simulink model "TASK1_regulation"  (R2024b)
settings: Solver=FixedStepAuto  StartTime=0.0  StopTime=inf  RelTol=1e-3
values from neighbouring files (symbols this model uses):
  D = diag([0.001, 0.001, 0.001, 0.0175/6, 0.0175/6, 0.0175/6*T_s, 0.0175/6*T_s].^2)    [TASK1_init_regulation.m]    (also in init_regulation.m)
  d = d_nominal    (= 0.165)    [TASK1_init_regulation.m]    (also in init_regulation.m)
  d_actual = d_nominal    (= 0.165)    [TASK1_init_regulation.m]    (also in init_regulation.m)
  omega_M = 10    [TASK1_init_regulation.m]    (also in init_regulation.m)
  P_INIT_EKF = diag([0.101, 0.101, 0.101, 0.0175/6, 0.0175/6, 0.0175/6*T_s, 0.0175/6*T_s].^2)    [TASK1_init_regulation.m]    (also in init_regulation.m = diag([0.001, 0.001, 0.001, 0.0175/6, 0.0175/6, 0.0175/6*T_s,)
  p_loss = 0    [TASK1_init_regulation.m]    (also in init_regulation.m)
  q_d = [x(2);y(2);0]    [TASK1_init_regulation.m]    (also in init_regulation.m = [2;2;0])
  Q_INIT = [x(1)+0.5;y(8)-0.5;-pi/2]    [TASK1_init_regulation.m]    (also in init_regulation.m = [0;0;0])
  r = r_nominal    (= 0.03)    [TASK1_init_regulation.m]    (also in init_regulation.m)
  R_2 = diag([ENCODER_QUANTIZATION/6,ENCODER_QUANTIZATION/6].^2)    [TASK1_init_regulation.m]    (also in init_regulation.m)
  R_3 = diag(([0.001, ENCODER_QUANTIZATION/6,ENCODER_QUANTIZATION/6]).^2)    [TASK1_init_regulation.m]    (also in init_regulation.m)
  R_4 = diag(([0.001, 0.001, ENCODER_QUANTIZATION/6,ENCODER_QUANTIZATION/6]).^2)    [TASK1_init_regulation.m]    (also in init_regulation.m)
  R_5 = diag(([0.001, 0.001, 0.001, ENCODER_QUANTIZATION/6,ENCODER_QUANTIZATION/6]).^2)    [TASK1_init_regulation.m]    (also in init_regulation.m)
  r_actual = r_nominal    (= 0.03)    [TASK1_init_regulation.m]    (also in init_regulation.m)
  T_s = 0.04    [TASK1_init_regulation.m]    (also in init_regulation.m)
  Z_INIT_EKF = [Q_INIT; 0; 0; 0; 0]    [TASK1_init_regulation.m]    (also in init_regulation.m)
undefined symbols (not defined in the file or in its folder): X, Y
libraries: robotlib x6, sharedtransform x1, dspsigops x1
settings Model: SimulationMode=external  Creator=riccardo01  LastModifiedBy=defendenri
settings DataIOCC: SaveFormat=Array  ReturnWorkspaceOutputs=off
settings OptimizationCC: DefaultParameterBehavior=Inlined  EnhancedBackFolding=on  PassReuseOutputArgsAs=Individual arguments  ZeroExternalMemoryAtStartup=off  ZeroInternalMemoryAtStartup=off  MaxStackSize=64  OptimizeBlockOrder=speed  DifferentSizesBufferReuse=on  OptimizationCustomize=off  EfficientTunableParamExpr=on
settings DebuggingCC: AlgebraicLoopMsg=none  ParameterTunabilityLossMsg=error
settings HardwareCC: ProdBitPerPointer=32  ProdBitPerSizeT=32  ProdBitPerPtrDiffT=32  ProdLargestAtomicFloat=None  ProdIntDivRoundTo=Undefined  ProdEndianess=Unspecified  ProdWordSize=32  ProdHWDeviceType=Generic->Unspecified (assume 32-bit Generic)
settings SFSimCC: MATLABDynamicMemAlloc=off
settings RTWCC: Description=Embedded Coder  SystemTargetFile=ert.tlc  HardwareBoard=Robot Operating System (ROS)  TLCOptions="-aInlineSetEventsForThisBaseRateFcn=TLC_FALSE -aSuppressMultiTaskScheduler=TLC_FALSE  -aRateBasedStepFcn=0"  TemplateMakefile=ert_default_tmf  Toolchain=Catkin  TargetLang=C++
settings CodeAppCC: ForceParamTrailComments=on  IgnoreCustomStorageClasses=off  OperatorAnnotations=on  SimulinkDataObjDesc=on  SFDataObjDesc=on  InsertBlockDesc=on

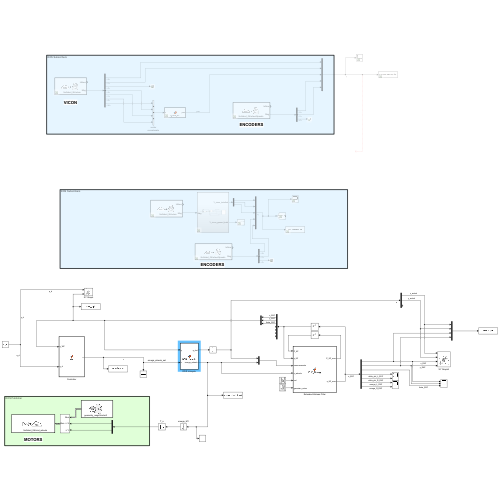
[thumbnail: Simulink's stored preview of the top-level diagram]
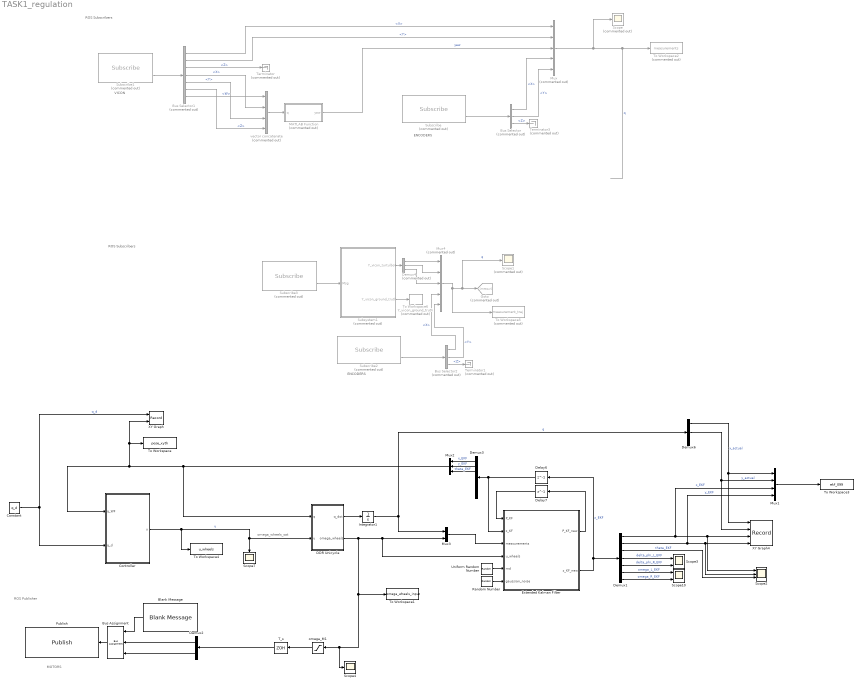
== system TASK1_regulation ==
  note: MOTORS
  note: ROS Publisher
  note: ENCODERS
  note: VICON
  note: ROS Subscribers
  note: omega_wheels_sat
  note: ENCODERS
  note: ROS Subscribers
  Blank Message : robotlib/Blank Message  messageClass=Message  entityType=geometry_msgs/Vector3  messageType=geometry_msgs/Vector3  SampleTime=T_s  legacyBusStruct=off
      settings: LibrarySourceBlock=roslib/ROS/Blank Message
  Bus Assignment : BusAssignment  AssignedSignals=X,Y
  Bus Selector : BusSelector  Commented=on  OutputSignals=X,Y,Z
  Bus Selector1 : BusSelector  Commented=on  OutputSignals=Pose.Pose.Position.X,Pose.Pose.Position.Y,Pose.Pose.Position.Z,Pose.Pose.Orientation.X,Pose.Pose.Orientation.Y,Pose.Pose.Orientation.Z,Pose.Pose.Orientation.W
  Bus Selector2 : BusSelector  Commented=on  OutputSignals=X,Y,Z
  Constant : Constant  Value=q_d
  Controller : MATLAB Function  TreatAsAtomicUnit=on
  DDR Unicycle : MATLAB Function  TreatAsAtomicUnit=on
  Delay6 : Delay  DelayLength=1  InitialCondition=Z_INIT_EKF  SampleTime=T_s
  Delay7 : Delay  DelayLength=1  InitialCondition=P_INIT_EKF  SampleTime=T_s
  Demux1 : Demux  Outputs=7
  Demux2 : Demux  Outputs=2
  Demux3 : Demux  Outputs=7
  Demux4 : Demux  Commented=on  Outputs=3
  Demux6 : Demux  Outputs=3
  Extended Kalman Filter : MATLAB Function  TreatAsAtomicUnit=on
  Goto : Goto  Commented=on  GotoTag=measur
  Integrator1 : Integrator  InitialCondition=Q_INIT
  MATLAB Function : MATLAB Function  Commented=on  TreatAsAtomicUnit=on
  Mux : Mux  Commented=on  Inputs=5
  Mux1 : Mux
  Mux2 : Mux  Inputs=3
  Mux3 : Mux  Inputs=2
  Mux4 : Mux  Commented=on  Inputs=5
  Publish : robotlib/Publish  topicSource=Specify your own  topic=/turtlebot_06/cmd_wheels  messageType=geometry_msgs/Vector3  legacyBusStruct=off  messageQueueLength=1
      settings: LibrarySourceBlock=roslib/ROS/Publish
  Random Number : RandomNumber  Variance=0.01  SampleTime=T_s
  Scope : Scope  Commented=on
  Scope1 : Scope  Commented=on
  Scope10 : Scope  NumInputPorts=2
  Scope2 : Scope  NumInputPorts=3
  Scope3 : Scope  NumInputPorts=2
  Scope4 : Scope
  Scope7 : Scope
  Subscribe : robotlib/Subscribe  Commented=on  topicSource=Specify your own  topic=/turtlebot_06/wheelSpeeds  messageType=geometry_msgs/Vector3  SampleTime=T_s  legacyBusStruct=off  messageQueueLength=1
      settings: LibrarySourceBlock=roslib/ROS/Subscribe
  Subscribe1 : robotlib/Subscribe  Commented=on  topicSource=Specify your own  topic=/turtlebot_06/odom  messageType=nav_msgs/Odometry  SampleTime=T_s  legacyBusStruct=off  messageQueueLength=1
      settings: LibrarySourceBlock=roslib/ROS/Subscribe
  Subscribe2 : robotlib/Subscribe  Commented=on  topicSource=Specify your own  topic=/turtlebot_06/wheelSpeeds  messageType=geometry_msgs/Vector3  SampleTime=T_s  legacyBusStruct=off  messageQueueLength=1
      settings: LibrarySourceBlock=roslib/ROS/Subscribe
  Subscribe3 : robotlib/Subscribe  Commented=on  topicSource=Specify your own  topic=/turtlebot_06/odom  messageType=nav_msgs/Odometry  SampleTime=T_s  legacyBusStruct=off  messageQueueLength=1
      settings: LibrarySourceBlock=roslib/ROS/Subscribe
  Subsystem1 : Subsystem  Commented=on
  T_s : ZeroOrderHold  SampleTime=T_s
  Terminator : Terminator  Commented=on
  Terminator1 : Terminator  Commented=on
  Terminator3 : Terminator  Commented=on
  To Workspace : ToWorkspace  VariableName=pose_xyth  SampleTime=-1
  To Workspace1 : ToWorkspace  VariableName=omega_wheels_input  SampleTime=-1
  To Workspace2 : ToWorkspace  Commented=on  VariableName=measurements  SampleTime=-1
  To Workspace3 : ToWorkspace  VariableName=ekf_099  SaveFormat=Structure With Time  SampleTime=-1
  To Workspace4 : ToWorkspace  VariableName=u_wheels  SampleTime=T_s
  To Workspace5 : ToWorkspace  Commented=on  VariableName=measurement_traj  SaveFormat=Timeseries  SampleTime=-1
  To Workspace6 : ToWorkspace  Commented=on  VariableName=Y_vicon_ground_truth  SaveFormat=Timeseries  SampleTime=T_s
  Uniform Random Number : UniformRandomNumber  Minimum=0  SampleTime=T_s
  XY Graph : Record  FileSettingsInternal="{\"entries\":[{\"content\":{\"excelSettings\":{\"content\":{},\"type\":\"Streamout.ExcelSettings\"}},\"type\":\"Streamout.FileSettingStorage\",\"uuid\":\"\"}],\"packageUris\":[\"http:\\/\\/schema.mathworks.com\\/mf0\\/streamout_blocks\\/R2020a\"],\"version\":\"1.0\"}"  Layout=[1 2]  SignalsInternal="{\"entries\":[{\"content\":{\"signals\":[{\"content\":{\"blockPath\":[],\"dimensions\":[3],\"domain\":\"\",\"hasChildren\":true,\"lineColor\":\"#7e2f8e\",\"lineWidth\":2,\"port\":2,\"sid\":[\"\"],\"signalID\":1,\"signalName\":\"Mux2\"},\"type\":\"RecordBlkView.Signal\",\"uuid\":\"\"},{\"content\":{\"blockPath\":[],\"channel\":[1],\"dimensions\":[3],\"domain\":\"\",\"lineColor\":\"#ff6929\",\"lineWidth\":2,\"parentID\":1,\"port\":2,\"sid\":[\"\"],\"signalID\":2,\"signalName\":\"Mux2\"},\"type\":\"RecordBlkView.Signal\",\"uuid\":\"\"},{\"content\":{\"blockPath\":[],\"dimensions\":[3],\"domain\":\"\",\"hasChildren\":true,\"lineColor\":\"#d95319\",\"lineWidth\":2,\"port\":1,\"sid\":[\"\"],\"signalID\":3,\"signalName\":\"q_d\"},\"type\":\"RecordBlkView.Signal\",\"uuid\":\"\"},{\"content\":{\"blockPath\":[],\"channel\":[1],\"dimensions\":[3],\"domain\":\"\",\"lineColor\":\"#a2142f\",\"lineWidth\":2,\"parentID\":3,\"port\":1,\"sid\":[\"\"],\"signalID\":4,\"signalName\":\"q_d\"},\"type\":\"RecordBlkView.Signal\",\"uuid\":\"\"},{\"content\":{\"blockPath\":[],\"channel\":[2],\"dimensions\":[3],\"domain\":\"\",\"lineColor\":\"#139fff\",\"lineWidth\":2,\"parentID\":1,\"port\":2,\"sid\":[\"\"],\"signalID\":5,\"signalName\":\"Mux2\"},\"type\":\"RecordBlkView.Signal\",\"uuid\":\"\"},{\"content\":{\"blockPath\":[],\"channel\":[3],\"dimensions\":[3],\"domain\":\"\",\"lineColor\":\"#ff6929\",\"lineWidth\":2,\"parentID\":1,\"port\":2,\"sid\":[\"\"],\"signalID\":6,\"signalName\":\"Mux2\"},\"type\":\"RecordBlkView.Signal\",\"uuid\":\"\"},{\"content\":{\"blockPath\":[],\"channel\":[2],\"dimensions\":[3],\"domain\":\"\",\"lineColor\":\"#d95319\",\"lineWidth\":2,\"parentID\":3,\"port\":1,\"sid\":[\"\"],\"signalID\":7,\"signalName\":\"q_d\"},\"type\":\"RecordBlkView.Signal\",\"uuid\":\"\"},{\"content\":{\"blockPath\":[],\"channel\":[3],\"dimensions\":[3],\"domain\":\"\",\"lineColor\":\"#edb120\",\"lineWidth\":2,\"parentID\":3,\"port\":1,\"sid\":[\"\"],\"signalID\":8,\"signalName\":\"q_d\"},\"type\":\"RecordBlkView.Signal\",\"uuid\":\"\"}]},\"type\":\"RecordBlkView.InputSignals\",\"uuid\":\"\"}],\"packageUris\":[\"http:\\/\\/schema.mathworks.com\\/mf0\\/streamout_blocks\\/R2020a\"],\"version\":\"1.0\"}"  VisualizationBindings="{\"xyplotplugin\":{\"info\":[{\"series\":[],\"subplotID\":1}]}}"  CompatibilityTag=XY
  XY Graph4 : Record  FileSettingsInternal="{\"entries\":[{\"content\":{\"excelSettings\":{\"content\":{},\"type\":\"Streamout.ExcelSettings\"}},\"type\":\"Streamout.FileSettingStorage\",\"uuid\":\"\"}],\"packageUris\":[\"http:\\/\\/schema.mathworks.com\\/mf0\\/streamout_blocks\\/R2020a\"],\"version\":\"1.0\"}"  Layout=[1 1]  SignalsInternal="{\"entries\":[{\"content\":{\"signals\":[{\"content\":{\"blockPath\":[],\"dimensions\":[1,1],\"domain\":\"\",\"lineColor\":\"#77ac30\",\"lineWidth\":2,\"plots\":[ 1 ],\"port\":1,\"sid\":[\"\"],\"signalID\":1,\"signalName\":\"x_actual\"},\"type\":\"RecordBlkView.Signal\",\"uuid\":\"\"},{\"content\":{\"blockPath\":[],\"dimensions\":[1,1],\"domain\":\"\",\"lineColor\":\"#4dbeee\",\"lineWidth\":2,\"plots\":[ 1 ],\"port\":2,\"sid\":[\"\"],\"signalID\":2,\"signalName\":\"y_actual\"},\"type\":\"RecordBlkView.Signal\",\"uuid\":\"\"},{\"content\":{\"blockPath\":[],\"dimensions\":[1],\"domain\":\"\",\"lineColor\":\"#a2142f\",\"lineWidth\":2,\"plots\":[ 1 ],\"port\":3,\"sid\":[\"\"],\"signalID\":3,\"signalName\":\"x_EKF\"},\"type\":\"RecordBlkView.Signal\",\"uuid\":\"\"},{\"content\":{\"blockPath\":[],\"dimensions\":[1],\"domain\":\"\",\"lineColor\":\"#139fff\",\"lineWidth\":2,\"plots\":[ 1 ],\"port\":4,\"sid\":[\"\"],\"signalID\":4,\"signalName\":\"y_EKF\"},\"type\":\"RecordBlkView.Signal\",\"uuid\":\"\"}]},\"type\":\"RecordBlkView.InputSignals\",\"uuid\":\"\"}],\"packageUris\":[\"http:\\/\\/schema.mathworks.com\\/mf0\\/streamout_blocks\\/R2020a\"],\"version\":\"1.0\"}"  VisualizationBindings="{\"xyplotplugin\":{\"info\":[{\"series\":[{\"bindingParametersList\":[{\"parameter\":\"X-Axis\",\"signalID\":3,\"signalName\":\"x_EKF\"},{\"parameter\":\"Y-Axis\",\"signalID\":4,\"signalName\":\"y_EKF\"}],\"seriesID\":0},{\"bindingParametersList\":[{\"parameter\":\"X-Axis\",\"signalID\":1,\"signalName\":\"x_actual\"},{\"parameter\":\"Y-Axis\",\"signalID\":2,\"signalName\":\"y_actual\"}],\"seriesID\":1}],\"subplotID\":1}]}}"  CompatibilityTag=XY
  omega_M1 : Saturate  UpperLimit=omega_M  LowerLimit=-omega_M
  vector concatenate : Concatenate  Commented=on  NumInputs=4
  wires:
  T_s/1 -> Demux2/1
  Blank Message/1 -> Bus Assignment/1
  Demux2/2 -> Bus Assignment/3
  Bus Assignment/1 -> Publish/1
  Demux2/1 -> Bus Assignment/2
  vector concatenate/1 -> MATLAB Function/1(q)
  Subscribe/2 -> Bus Selector/1
  Bus Selector1/5 -> vector concatenate/3  "<Y>"
  Bus Selector/2 -> Mux/5  "<Y>"
  Bus Selector1/3 -> Terminator/1  "<Z>"
  Bus Selector1/1 -> Mux/1  "<X>"
  MATLAB Function/1(yaw) -> Mux/3  "yaw"
  Subscribe1/2 -> Bus Selector1/1
  Bus Selector1/6 -> vector concatenate/4  "<Z>"
  Bus Selector/1 -> Mux/4  "<X>"
  Mux/1 -> Scope/1, To Workspace2/1  "q"
  Bus Selector/3 -> Terminator3/1  "<Z>"
  Bus Selector1/2 -> Mux/2  "<Y>"
  Bus Selector1/7 -> vector concatenate/1  "<W>"
  Bus Selector1/4 -> vector concatenate/2  "<X>"
  Controller/1(u) -> To Workspace4/1, DDR Unicycle/2(u), Scope7/1  "u"
  DDR Unicycle/1(q_dot) -> Integrator1/1
  Constant/1 -> Controller/2(q_d), XY Graph/1  "q_d"
  Demux1/4 -> Scope3/1  "delta_phi_L_EKF"
  Demux6/1 -> Mux1/1, XY Graph4/1  "x_actual"
  Demux1/5 -> Scope3/2  "delta_phi_R_EKF"
  Delay6/1 -> Demux3/1, Extended Kalman Filter/2(z_KF)
  Random Number/1 -> Extended Kalman Filter/6(gaussian_noise)
  Mux1/1 -> To Workspace3/1
  Integrator1/1 -> Demux6/1, Mux3/1  "q"
  Extended Kalman Filter/1(P_KF_new) -> Delay7/1
  Demux1/2 -> Mux1/4, Scope2/2, XY Graph4/4  "y_EKF"
  Demux6/2 -> Mux1/2, XY Graph4/2  "y_actual"
  Delay7/1 -> Extended Kalman Filter/1(P_KF)
  Extended Kalman Filter/2(z_KF_new) -> Demux1/1, Delay6/1  "z_EKF"
  Demux1/3 -> Scope2/3  "theta_EKF"
  Demux1/7 -> Scope10/2  "omega_R_EKF"
  Demux1/6 -> Scope10/1  "omega_L_EKF"
  Uniform Random Number/1 -> Extended Kalman Filter/5(rnd)
  Demux1/1 -> Mux1/3, Scope2/1, XY Graph4/3  "x_EKF"
  omega_M1/1 -> T_s/1
  DDR Unicycle/2(omega_wheels) -> Extended Kalman Filter/4(u_wheels), Mux3/2, To Workspace1/1, Scope4/1, omega_M1/1
  Demux3/1 -> Mux2/1  "x_EKF"
  Demux3/2 -> Mux2/2  "y_EKF"
  Demux3/3 -> Mux2/3  "theta_EKF"
  Mux3/1 -> Extended Kalman Filter/3(messurements)
  Mux2/1 -> DDR Unicycle/1(q), Controller/1(q_WF), XY Graph/2, To Workspace/1
  Mux4/1 -> To Workspace5/1, Goto/1, Scope1/1  "q"
  Demux4/2 -> Mux4/2
  Subscribe3/2 -> Subsystem1/1(Msg)
  Demux4/1 -> Mux4/1
  Subscribe2/2 -> Bus Selector2/1
  Bus Selector2/2 -> Mux4/5  "<Y>"
  Bus Selector2/1 -> Mux4/4  "<X>"
  Demux4/3 -> Mux4/3
  Subsystem1/1(Y_vicon_turtulbot) -> Demux4/1
  Bus Selector2/3 -> Terminator1/1  "<Z>"
  Subsystem1/2(Y_vicon_ground_truth) -> To Workspace6/1

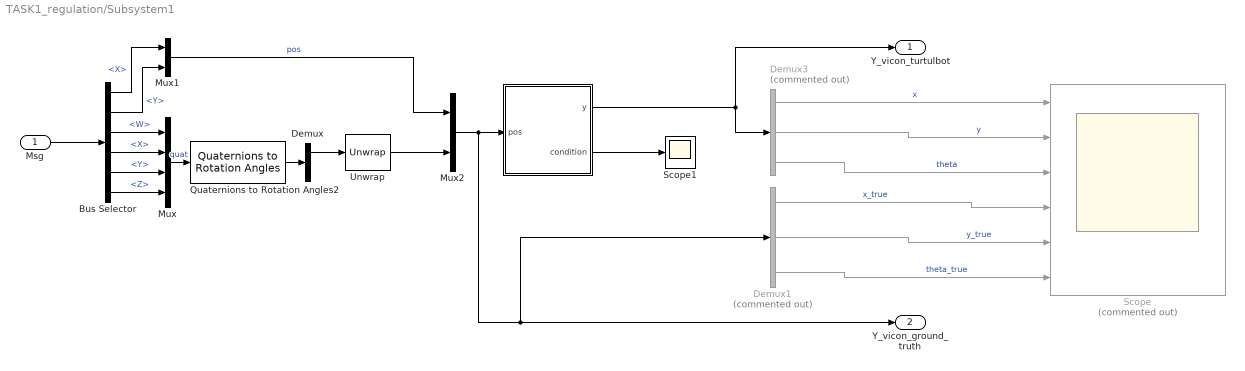
== system TASK1_regulation/Subsystem1 ==
  Msg : Inport
  " " : MATLAB Function  TreatAsAtomicUnit=on
  Bus Selector : BusSelector  OutputSignals=Pose.Pose.Position.X,Pose.Pose.Position.Y,Pose.Pose.Orientation.W,Pose.Pose.Orientation.X,Pose.Pose.Orientation.Y,Pose.Pose.Orientation.Z
  Demux : Demux  Outputs=3
  Demux1 : Demux  Commented=on  Outputs=3
  Demux3 : Demux  Commented=on  Outputs=3
  Mux : Mux
  Mux1 : Mux  Inputs=2
  Mux2 : Mux  Inputs=2
  Quaternions to Rotation Angles2 : sharedtransform/Quaternions to Rotation Angles  rotationOrder=ZYX  aMode=aMode
  Scope : Scope  Commented=on  NumInputPorts=6
  Scope1 : Scope
  Unwrap : dspsigops/Unwrap  tol=pi  InputProcessing=Columns as channels (frame based)  running=off
  Y_vicon_turtulbot : Outport
  Y_vicon_ground_truth : Outport  Port=2
  wires:
  Demux/1 -> Unwrap/1
  Quaternions to Rotation Angles2/1 -> Demux/1
  Mux1/1 -> Mux2/1  "pos"
  Unwrap/1 -> Mux2/2
  Demux1/1 -> Scope/4  "x_true"
  Demux3/2 -> Scope/2  "y"
  Demux3/3 -> Scope/3  "theta"
  " "/2(condition) -> Scope1/1
  Demux1/3 -> Scope/6  "theta_true"
  Bus Selector/5 -> Mux/3  "<Y>"
  Bus Selector/4 -> Mux/2  "<X>"
  Demux1/2 -> Scope/5  "y_true"
  " "/1(y) -> Demux3/1, Y_vicon_turtulbot/1
  Bus Selector/1 -> Mux1/1  "<X>"
  Bus Selector/6 -> Mux/4  "<Z>"
  Demux3/1 -> Scope/1  "x"
  Bus Selector/2 -> Mux1/2  "<Y>"
  Mux/1 -> Quaternions to Rotation Angles2/1  "quat"
  Bus Selector/3 -> Mux/1  "<W>"
  Mux2/1 -> " "/1(pos), Y_vicon_ground_truth/1, Demux1/1
  Msg/1 -> Bus Selector/1

== matlab function TASK1_regulation/Controller ==
  data: q_WF input; q_d input; u output; control_par parameter
function u = fcn(q_WF, q_d, control_par)

% roto translation
omega_d = q_d(3);
e = q_WF - q_d;
q_WF(1) = cos(omega_d)*e(1) + sin(omega_d)*e(2);
q_WF(2) = -sin(omega_d)*e(1) + cos(omega_d)*e(2);
q_WF(3) = e(3);


% posture regulator
% transform q_WF
% compute pointing error

ro = sqrt(q_WF(1)^2 + q_WF(2)^2);
% pointing error
gamma = wrapToPi(atan2(q_WF(2),q_WF(1)) + pi - q_WF(3));
delta = wrapToPi(gamma + q_WF(3));

v = control_par(1) * ro * cos(gamma);

if abs(gamma)<1e-4
    omega = control_par(2)*gamma + control_par(1)*cos(gamma)*(gamma + control_par(3)*delta);
else
    omega = control_par(2)*gamma + control_par(1)*sin(gamma)*cos(gamma)*(gamma + control_par(3)*delta)/gamma;
end

u = [v;omega];

== matlab function TASK1_regulation/DDR Unicycle ==
  data: q input; u input; q_dot output; omega_wheels output; d_actual parameter; r_actual parameter; omega_M parameter
function [q_dot,  omega_wheels]  = DDR_Unicycle(q, u, d_actual, r_actual, omega_M)

omega_wheels = [u(1)/r_actual - d_actual*u(2)/(2*r_actual);
                u(1)/r_actual + d_actual*u(2)/(2*r_actual)];

q_dot = [cos(q(3))*u(1);
         sin(q(3))*u(1);
         u(2)];


% PROPORTIONAL SATURATION 
if (abs(omega_wheels(1)) > omega_M) || (abs(omega_wheels(2)) > omega_M)
    omega_prop = max(abs(omega_wheels(1)), abs(omega_wheels(2)));
    omega_wheels(1) = omega_wheels(1)*omega_M/omega_prop;
    omega_wheels(2) = omega_wheels(2)*omega_M/omega_prop;
end

end

== matlab function TASK1_regulation/Subsystem1/  ==
  data: y output; pos input; condition output
function [y, condition] = check(pos)

x1 = -2.9; y1 = -1.5;
x2 = -1.6; y2 = -1.1;
x3 = -1.5; y3 = -0.7;
x4 = -1.4; y4 = -0.3;
x5 = -0.6; y5 =  0.1;
x6 =  0.2; y6 =  1.5;
x7 =  1.0;
x8 =  1.1;
x9 =  2.9;

P_loss = 0.9;


if ((pos(1) >= x5) && (pos(1) <= x6)) && ((pos(2) >= y1) && (pos(2) <= y5))
    % add noise
    y = pos + 0.02*randn(3,1);
    condition = 1;
elseif ((pos(1) >= x7) && (pos(1) <= x9)) && ((pos(2) >= y1) && (pos(2) <= y6))
    % measurement loss
    if rand > P_loss
        y = pos;
    else
        y = 0*pos;
    end
    condition = 2;
else
    y = pos;
    condition = 0;
end

== matlab function TASK1_regulation/Extended Kalman Filter ==
  data: P_KF input; P_KF_new output; z_KF input; messurements input; z_KF_new output; u_wheels input; D parameter; R_2 parameter; R_3 parameter; R_4 parameter; R_5 parameter; T_s parameter; r parameter; d parameter; p_loss parameter; rnd input; gaussian_noise input
function [P_KF_new, z_KF_new] = EKF_filtering(P_KF, z_KF, messurements, u_wheels, D, R_2, R_3, R_4, R_5 ,T_s, r, d, p_loss, rnd, gaussian_noise)

% z_KF = [x_EKF, y_EKF, theta_EKF, delta_phi_L_EKF, delta_phi_R_EKF, omega_L_EKF, omega_R_EKF]

v_k = r * (z_KF(6) + z_KF(7))/2;
w_k = r * (z_KF(7) - z_KF(6))/d;
theta_mean = z_KF(3) + (w_k * T_s)/2;

F_k = [1, 0, -T_s * v_k * sin(theta_mean), 0, 0, T_s * r * cos(theta_mean)/2 + (T_s)^2 * r * v_k * sin(theta_mean)/(2*d), T_s * r * cos(theta_mean)/2 - (T_s)^2 * r * v_k * sin(theta_mean)/(2*d);
       0, 1,  T_s * v_k * cos(theta_mean), 0, 0, T_s * r * sin(theta_mean)/2 - (T_s)^2 * r * v_k * cos(theta_mean)/(2*d), T_s * r * sin(theta_mean)/2 + (T_s)^2 * r * v_k * cos(theta_mean)/(2*d);
       0, 0, 1, 0, 0, (-T_s*r)/d, (T_s*r)/d;
       0, 0, 0, 0, 0, T_s, 0;
       0, 0, 0, 0, 0, 0, T_s;
       0, 0, 0, 0, 0, 0, 0;
       0, 0, 0, 0, 0, 0, 0];

%% Prediction part

z_pred = [z_KF(1)+(T_s*r*(z_KF(6)+z_KF(7))/2)*cos(theta_mean + (T_s*r*(z_KF(6)+z_KF(7)))/(2*d)); 
          z_KF(2)+(T_s*r*(z_KF(6)+z_KF(7))/2)*sin(theta_mean + (T_s*r*(z_KF(7)-z_KF(6)))/(2*d));
          theta_mean + (T_s*r*(z_KF(7)-z_KF(6))/(2*d));
          T_s*z_KF(6);
          T_s*z_KF(7);
          u_wheels(1);
          u_wheels(2)];

P_pred = F_k * P_KF * F_k' + D;


%% Update

%%if(rnd<p_loss) 
if(true)
    % Just encoders
    y_messurement = [messurements(1); messurements(2)];
    H = [0, 0, 0, 0, 0, 1, 0;
         0, 0, 0, 0, 0, 0, 1];

    e = y_messurement - H * z_pred;
    K = P_pred * H' /(H * P_pred * H' + R_2);

    z_KF_new = z_pred +  K * e;
    P_KF_new = P_pred - K * H * P_pred;

else 
    % GPS(x,y) + Encoders
    y_messurement = [messurements(1)+gaussian_noise;messurements(2)+gaussian_noise; messurements(3)+gaussian_noise;messurements(4); messurements(5)];

    H = [1, 0, 0, 0, 0, 0, 0;
         0, 1, 0, 0, 0, 0, 0;
         0, 0, 1, 0, 0, 0, 0;
         0, 0, 0, 0, 0, 1, 0;
         0, 0, 0, 0, 0, 0, 1];

    e = y_messurement - H * z_pred;
    K = P_pred * H' /(H * P_pred * H' + R_5);

    z_KF_new = z_pred + K * e;
    P_KF_new = P_pred - K * H * P_pred;

end

== matlab function TASK1_regulation/MATLAB Function ==
  data: q input; yaw output
function yaw = quat2yaw(q)

% normalize to avoid issues
q = q / norm(q);

w = q(1);
x = q(2);
y = q(3);
z = q(4);

% rotation around Z axis
yaw = atan2(2*(w*z + x*y), 1 - 2*(y^2 + z^2));

end
